simulink model "modelosanfis"  (R2017a)
settings: Solver=VariableStepAuto  StartTime=0.0  StopTime=578  RelTol=1e-3  EnableMultiTasking=on
values from neighbouring files (symbols this model uses):
  dinneg12 = [-0.01 -0.01 -0.02 -0.01 -0.01 -0.01 0 0 0 0 0.01 -0.01 ... (2312 elements, 578x4)]    [anfisd.mat]    (also in anfisfin.mat; cinco.mat)
  dinnegc12 = [-0.01 -0.01 -0.02 -0.01 -0.01 -0.01 0 0 0 0 0.01 -0.01 ... (2312 elements, 578x4)]    [anfisd.mat]    (also in anfisfin.mat; cinco.mat)
  dinpos12 = [0 0 0 0 0 0.01 0.01 0.01 0.01 0.01 0.01 0.01 ... (2400 elements, 600x4)]    [anfisd.mat]    (also in anfisfin.mat; cinco.mat)
  dinpos12c = [0 0 0 0 0 0.01 0.01 0.01 0.01 0.01 0.01 0.01 ... (2400 elements, 600x4)]    [anfisd.mat]    (also in anfisfin.mat; cinco.mat)
libraries: dspsrcs4 x37, fuzblock x13, simulink x2
settings Model: Creator=70459  LastModifiedBy=Dell
settings OptimizationCC: LifeSpan=inf
settings DebuggingCC: SFUnexpectedBacktrackingDiag=warning  SFNoUnconditionalDefaultTransitionDiag=warning  SFExecutionAtInitializationDiag=none
settings GRTTargetCC: TargetLangStandard=C89/C90 (ANSI)  GeneratePreprocessorConditionals=Disable all
settings ConfigComp: CovMetricSettings=dw  CovHtmlReporting=on  CovSaveCumulativeToWorkspaceVar=on  CovSaveSingleToWorkspaceVar=on  CovExternalEMLEnable=off

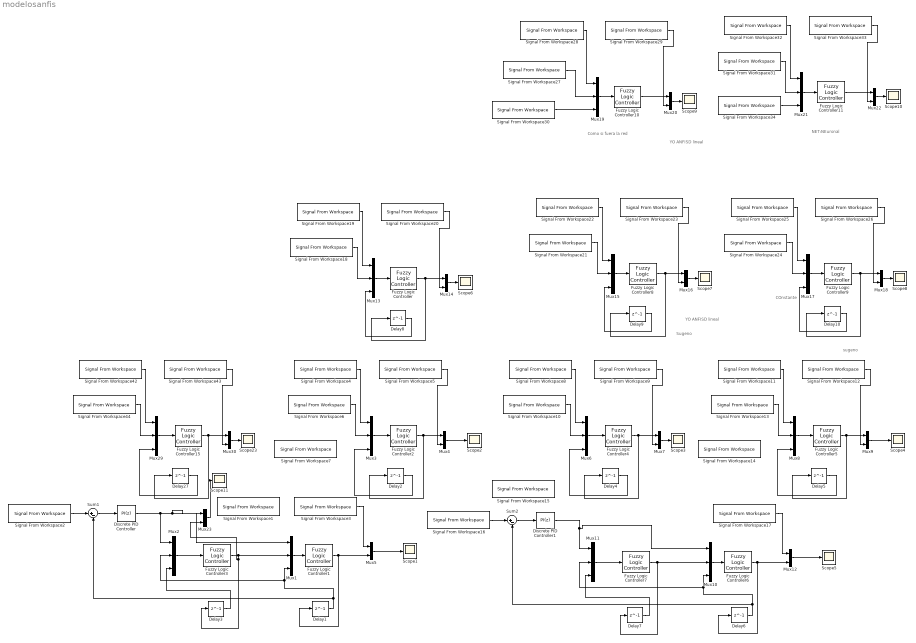
== system modelosanfis ==
  note: NET:NEuronal
  note: Como si fuera la red
  note: sugeno
  note: Sugeno
  note: COnstante
  note: YO ANFISD lineal
  note: YO ANFISD lineal
  Delay{1..10,27} (11 alike) : Delay  DelayLength=1
  Discrete PID Controller : simulink/Continuous/PID Controller  Controller=PI  TimeDomain=Discrete-time  SampleTime=1  IntegratorMethod=Forward Euler  FilterMethod=Forward Euler  Form=Parallel  UseFilter=on  ControllerParametersSource=internal  P=0.0433317577986285  I=0.000198935432291646  D=0  N=100  InitialConditionSource=internal  InitialConditionForIntegrator=0  InitialConditionForFilter=0  ExternalReset=none  LimitOutput=on  UpperSaturationLimit=1  LowerSaturationLimit=-1  LinearizeAsGain=off  AntiWindupMode=none  Kb=1  TrackingMode=off  Kt=1  PParamMin=[]  PParamMax=[]  IParamMin=[]  IParamMax=[]  DParamMin=[]  DParamMax=[]  NParamMin=[]  NParamMax=[]  KbParamMin=[]  KbParamMax=[]  KtParamMin=[]  KtParamMax=[]  POutMin=[]  POutMax=[]  IOutMin=[]  IOutMax=[]  DOutMin=[]  DOutMax=[]  NOutMin=[]  NOutMax=[]  KbOutMin=[]  KbOutMax=[]  KtOutMin=[]  KtOutMax=[]  IntegratorOutMin=[]  IntegratorOutMax=[]  FilterOutMin=[]  FilterOutMax=[]  SumOutMin=[]  SumOutMax=[]  SumI1OutMin=[]  SumI1OutMax=[]  SumI2OutMin=[]  SumI2OutMax=[]  SumI3OutMin=[]  SumI3OutMax=[]  SumDOutMin=[]  SumDOutMax=[]  SaturationOutMin=[]  SaturationOutMax=[]  IntegratorContinuousStateAttributes=''  IntegratorStateMustResolveToSignalObject=off  IntegratorRTWStateStorageClass=Auto  FilterContinuousStateAttributes=''  FilterStateMustResolveToSignalObject=off  FilterRTWStateStorageClass=Auto  DifferentiatorICPrevScaledInput=0  DifferentiatorOutMin=[]  DifferentiatorOutMax=[]  InitialConditionSetting=State (most efficient)
  Discrete PID Controller1 : simulink/Continuous/PID Controller  Controller=PI  TimeDomain=Discrete-time  SampleTime=1  IntegratorMethod=Forward Euler  FilterMethod=Forward Euler  Form=Parallel  UseFilter=on  ControllerParametersSource=internal  P=0.0396555203379385  I=0.0007259172184210663  D=0  N=100  InitialConditionSource=internal  InitialConditionForIntegrator=0  InitialConditionForFilter=0  ExternalReset=none  LimitOutput=on  UpperSaturationLimit=1  LowerSaturationLimit=-1  LinearizeAsGain=off  AntiWindupMode=none  Kb=1  TrackingMode=off  Kt=1  PParamMin=[]  PParamMax=[]  IParamMin=[]  IParamMax=[]  DParamMin=[]  DParamMax=[]  NParamMin=[]  NParamMax=[]  KbParamMin=[]  KbParamMax=[]  KtParamMin=[]  KtParamMax=[]  POutMin=[]  POutMax=[]  IOutMin=[]  IOutMax=[]  DOutMin=[]  DOutMax=[]  NOutMin=[]  NOutMax=[]  KbOutMin=[]  KbOutMax=[]  KtOutMin=[]  KtOutMax=[]  IntegratorOutMin=[]  IntegratorOutMax=[]  FilterOutMin=[]  FilterOutMax=[]  SumOutMin=[]  SumOutMax=[]  SumI1OutMin=[]  SumI1OutMax=[]  SumI2OutMin=[]  SumI2OutMax=[]  SumI3OutMin=[]  SumI3OutMax=[]  SumDOutMin=[]  SumDOutMax=[]  SaturationOutMin=[]  SaturationOutMax=[]  IntegratorContinuousStateAttributes=''  IntegratorStateMustResolveToSignalObject=off  IntegratorRTWStateStorageClass=Auto  FilterContinuousStateAttributes=''  FilterStateMustResolveToSignalObject=off  FilterRTWStateStorageClass=Auto  DifferentiatorICPrevScaledInput=0  DifferentiatorOutMin=[]  DifferentiatorOutMax=[]  InitialConditionSetting=State (most efficient)
  Fuzzy Logic Controller : fuzblock/Fuzzy Logic  Controller  fis=ANFISD
  Fuzzy Logic Controller1 : fuzblock/Fuzzy Logic  Controller  fis=anfisd12
  Fuzzy Logic Controller10 : fuzblock/Fuzzy Logic  Controller  fis=ANFISD
  Fuzzy Logic Controller11 : fuzblock/Fuzzy Logic  Controller  fis=ANFISDC1
  Fuzzy Logic Controller15 : fuzblock/Fuzzy Logic  Controller  fis=anfisd12
  Fuzzy Logic Controller2 : fuzblock/Fuzzy Logic  Controller  fis=anfisd12c
  Fuzzy Logic Controller3 : fuzblock/Fuzzy Logic  Controller  fis=anfisd12c
  Fuzzy Logic Controller4 : fuzblock/Fuzzy Logic  Controller  fis=anfisneg12
  Fuzzy Logic Controller5 : fuzblock/Fuzzy Logic  Controller  fis=anfis1222
  Fuzzy Logic Controller6 : fuzblock/Fuzzy Logic  Controller  fis=anfisneg12
  Fuzzy Logic Controller7 : fuzblock/Fuzzy Logic  Controller  fis=anfis1222
  Fuzzy Logic Controller8 : fuzblock/Fuzzy Logic  Controller  fis=ANFISD
  Fuzzy Logic Controller9 : fuzblock/Fuzzy Logic  Controller  fis=ANFISDC1
  Mux{1..3,6,8,10..11,13,15,17,19,21,29} (13 alike) : Mux  Inputs=3
  Mux{4..5,7,9,12,14,16,18,20,22..23,30} (12 alike) : Mux  Inputs=2
  Scope{1..11,23} (12 alike) : Scope
  Signal From Workspace{1,4,7,14} (4 alike) : dspsrcs4/Signal From Workspace  X=dinpos12c(:,1)  Ts=1  nsamps=1  OutputAfterFinalValue=Setting to zero  ignoreOrWarnInputAndFrameLengths=off  OutputFrames=off
  Signal From Workspace{10,18,21,24,27,31} (6 alike) : dspsrcs4/Signal From Workspace  X=dinneg12(:,2)  Ts=1  nsamps=1  OutputAfterFinalValue=Setting to zero  ignoreOrWarnInputAndFrameLengths=off  OutputFrames=off
  Signal From Workspace11 : dspsrcs4/Signal From Workspace  X=dinnegc12(:,1)  Ts=1  nsamps=1  OutputAfterFinalValue=Setting to zero  ignoreOrWarnInputAndFrameLengths=off  OutputFrames=off
  Signal From Workspace12 : dspsrcs4/Signal From Workspace  X=dinnegc12(:,4)  Ts=1  nsamps=1  OutputAfterFinalValue=Setting to zero  ignoreOrWarnInputAndFrameLengths=off  OutputFrames=off
  Signal From Workspace13 : dspsrcs4/Signal From Workspace  X=dinnegc12(:,2)  Ts=1  nsamps=1  OutputAfterFinalValue=Setting to zero  ignoreOrWarnInputAndFrameLengths=off  OutputFrames=off
  Signal From Workspace{8,15,19,22,25,28,32} (7 alike) : dspsrcs4/Signal From Workspace  X=dinneg12(:,1)  Ts=1  nsamps=1  OutputAfterFinalValue=Setting to zero  ignoreOrWarnInputAndFrameLengths=off  OutputFrames=off
  Signal From Workspace16 : dspsrcs4/Signal From Workspace  X=ref2  Ts=1  nsamps=1  OutputAfterFinalValue=Setting to zero  ignoreOrWarnInputAndFrameLengths=off  OutputFrames=off
  Signal From Workspace17 : dspsrcs4/Signal From Workspace  X=ref2  Ts=1  nsamps=1  OutputAfterFinalValue=Setting to zero  ignoreOrWarnInputAndFrameLengths=off  OutputFrames=off
  Signal From Workspace2 : dspsrcs4/Signal From Workspace  X=ref  Ts=1  nsamps=1  OutputAfterFinalValue=Setting to zero  ignoreOrWarnInputAndFrameLengths=off  OutputFrames=off
  Signal From Workspace{9,20,23,26,29,33} (6 alike) : dspsrcs4/Signal From Workspace  X=dinneg12(:,4)  Ts=1  nsamps=1  OutputAfterFinalValue=Setting to zero  ignoreOrWarnInputAndFrameLengths=off  OutputFrames=off
  Signal From Workspace3 : dspsrcs4/Signal From Workspace  X=ref  Ts=1  nsamps=1  OutputAfterFinalValue=Setting to zero  ignoreOrWarnInputAndFrameLengths=off  OutputFrames=off
  Signal From Workspace30 : dspsrcs4/Signal From Workspace  X=dinneg12(:,3)  Ts=1  nsamps=1  OutputAfterFinalValue=Setting to zero  ignoreOrWarnInputAndFrameLengths=off  OutputFrames=off
  Signal From Workspace34 : dspsrcs4/Signal From Workspace  X=dinneg12(:,3)  Ts=1  nsamps=1  OutputAfterFinalValue=Setting to zero  ignoreOrWarnInputAndFrameLengths=off  OutputFrames=off
  Signal From Workspace42 : dspsrcs4/Signal From Workspace  X=dinpos12(:,1)  Ts=1  nsamps=1  OutputAfterFinalValue=Setting to zero  ignoreOrWarnInputAndFrameLengths=off  OutputFrames=off
  Signal From Workspace43 : dspsrcs4/Signal From Workspace  X=dinpos12(:,4)  Ts=1  nsamps=1  OutputAfterFinalValue=Setting to zero  ignoreOrWarnInputAndFrameLengths=off  OutputFrames=off
  Signal From Workspace44 : dspsrcs4/Signal From Workspace  X=dinpos12(:,2)  Ts=1  nsamps=1  OutputAfterFinalValue=Setting to zero  ignoreOrWarnInputAndFrameLengths=off  OutputFrames=off
  Signal From Workspace5 : dspsrcs4/Signal From Workspace  X=dinpos12c(:,4)  Ts=1  nsamps=1  OutputAfterFinalValue=Setting to zero  ignoreOrWarnInputAndFrameLengths=off  OutputFrames=off
  Signal From Workspace6 : dspsrcs4/Signal From Workspace  X=dinpos12c(:,2)  Ts=1  nsamps=1  OutputAfterFinalValue=Setting to zero  ignoreOrWarnInputAndFrameLengths=off  OutputFrames=off
  Sum1 : Sum  Inputs=|+-
  Sum2 : Sum  Inputs=|+-
  wires:
  Mux29/1 -> Fuzzy Logic Controller15/1
  Fuzzy Logic Controller15/1 -> Delay27/1, Mux30/1
  Mux30/1 -> Scope23/1
  Signal From Workspace42/1 -> Mux29/1
  Signal From Workspace43/1 -> Mux30/2
  Delay27/1 -> Mux29/3
  Signal From Workspace44/1 -> Mux29/2
  Mux3/1 -> Fuzzy Logic Controller2/1
  Fuzzy Logic Controller2/1 -> Delay2/1, Mux4/1
  Delay2/1 -> Mux3/3
  Mux4/1 -> Scope2/1
  Signal From Workspace4/1 -> Mux3/1
  Signal From Workspace5/1 -> Mux4/2
  Signal From Workspace6/1 -> Mux3/2
  Mux1/1 -> Fuzzy Logic Controller1/1
  Fuzzy Logic Controller3/1 -> Mux23/2, Delay3/1, Mux1/2
  Mux2/1 -> Fuzzy Logic Controller3/1
  Fuzzy Logic Controller1/1 -> Mux5/2, Delay1/1
  Delay1/1 -> Mux2/2, Mux1/3, Sum1/2
  Delay3/1 -> Mux2/3
  Mux5/1 -> Scope1/1
  Signal From Workspace3/1 -> Mux5/1
  Sum1/1 -> Discrete PID Controller/1
  Signal From Workspace2/1 -> Sum1/1
  Mux6/1 -> Fuzzy Logic Controller4/1
  Fuzzy Logic Controller4/1 -> Delay4/1, Mux7/1
  Mux7/1 -> Scope3/1
  Signal From Workspace8/1 -> Mux6/1
  Signal From Workspace9/1 -> Mux7/2
  Delay4/1 -> Mux6/3
  Signal From Workspace10/1 -> Mux6/2
  Mux8/1 -> Fuzzy Logic Controller5/1
  Fuzzy Logic Controller5/1 -> Delay5/1, Mux9/1
  Delay5/1 -> Mux8/3
  Mux9/1 -> Scope4/1
  Signal From Workspace11/1 -> Mux8/1
  Signal From Workspace12/1 -> Mux9/2
  Signal From Workspace13/1 -> Mux8/2
  Mux10/1 -> Fuzzy Logic Controller6/1
  Fuzzy Logic Controller7/1 -> Delay7/1, Mux10/2
  Mux11/1 -> Fuzzy Logic Controller7/1
  Fuzzy Logic Controller6/1 -> Mux12/2, Delay6/1
  Delay6/1 -> Mux11/2, Mux10/3, Sum2/2
  Delay7/1 -> Mux11/3
  Mux12/1 -> Scope5/1
  Signal From Workspace17/1 -> Mux12/1
  Sum2/1 -> Discrete PID Controller1/1
  Signal From Workspace16/1 -> Sum2/1
  Discrete PID Controller1/1 -> Mux10/1, Mux11/1
  Signal From Workspace18/1 -> Mux13/2
  Delay8/1 -> Mux13/3
  Signal From Workspace20/1 -> Mux14/2
  Signal From Workspace19/1 -> Mux13/1
  Mux14/1 -> Scope6/1
  Fuzzy Logic Controller/1 -> Delay8/1, Mux14/1
  Mux13/1 -> Fuzzy Logic Controller/1
  Mux15/1 -> Fuzzy Logic Controller8/1
  Fuzzy Logic Controller8/1 -> Mux16/1, Delay9/1
  Mux16/1 -> Scope7/1
  Signal From Workspace22/1 -> Mux15/1
  Signal From Workspace23/1 -> Mux16/2
  Delay9/1 -> Mux15/3
  Signal From Workspace21/1 -> Mux15/2
  Signal From Workspace24/1 -> Mux17/2
  Delay10/1 -> Mux17/3
  Signal From Workspace26/1 -> Mux18/2
  Signal From Workspace25/1 -> Mux17/1
  Mux18/1 -> Scope8/1
  Fuzzy Logic Controller9/1 -> Delay10/1, Mux18/1
  Mux17/1 -> Fuzzy Logic Controller9/1
  Mux19/1 -> Fuzzy Logic Controller10/1
  Signal From Workspace29/1 -> Mux20/2
  Mux20/1 -> Scope9/1
  Signal From Workspace28/1 -> Mux19/1
  Fuzzy Logic Controller10/1 -> Mux20/1
  Signal From Workspace27/1 -> Mux19/2
  Signal From Workspace30/1 -> Mux19/3
  Mux21/1 -> Fuzzy Logic Controller11/1
  Fuzzy Logic Controller11/1 -> Mux22/1
  Mux22/1 -> Scope10/1
  Signal From Workspace32/1 -> Mux21/1
  Signal From Workspace33/1 -> Mux22/2
  Signal From Workspace31/1 -> Mux21/2
  Signal From Workspace34/1 -> Mux21/3
  Discrete PID Controller/1 -> Mux23/1, Mux1/1, Mux2/1
  Mux23/1 -> Scope11/1
